simulink model "Buck_Converter_with_3ph_Full_Bridge_Rectifier"  (R2022b)
settings: Solver=VariableStepAuto  StartTime=0.0  StopTime=1.5  RelTol=1e-3
libraries: spsDiodeLib x7, spsSeriesRLCBranchLib x6, spsRMSLib x4, spsVoltageMeasurementLib x3, slpidlib x1, simulink x1, spsCurrentMeasurementLib x1, spsGroundLib x1, spsDCMachineLib x1, spsDCVoltageSourceLib x1, spsIGBTDiodeLib x1, spsPower3phInstantaneousLib x1
settings Model: Creator=meteh  LastModifiedBy=meteh
settings SolverCC: ZeroCrossAlgorithm=Adaptive
settings DebuggingCC: IgnoredZcDiagnostic=none

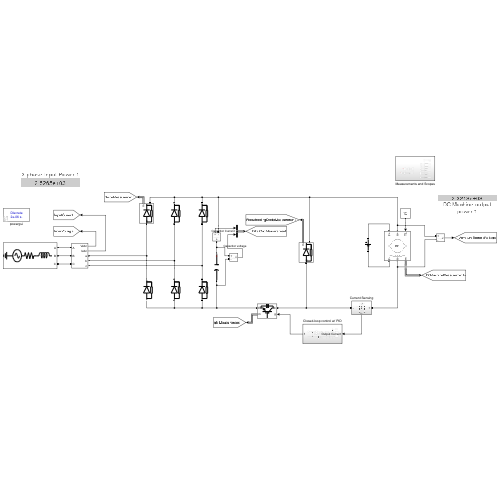
[thumbnail: Simulink's stored preview of the top-level diagram]
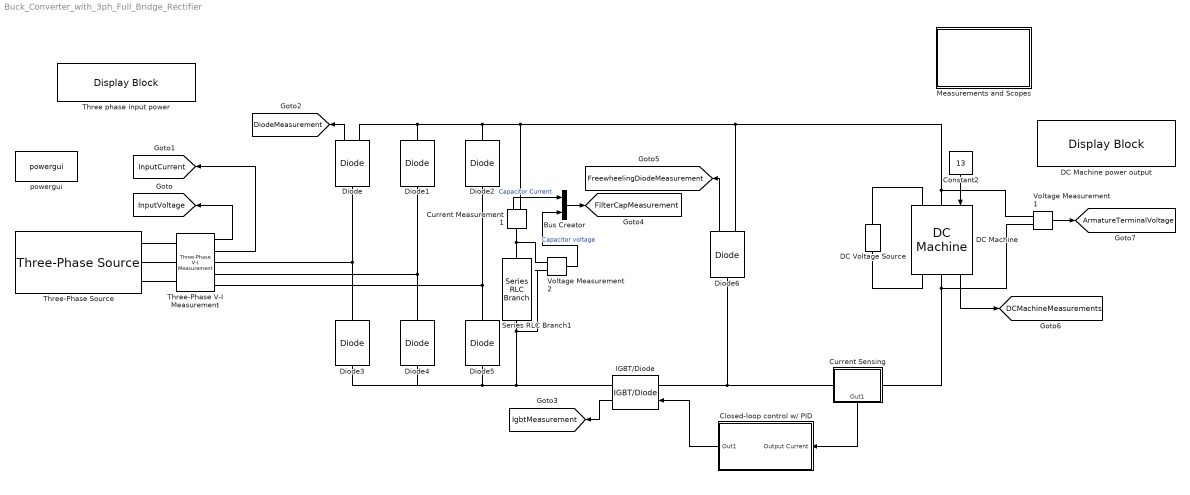
== system Buck_Converter_with_3ph_Full_Bridge_Rectifier ==
  Bus Creator : BusCreator  Inputs=2
  Closed-loop control w/ PID : Subsystem
  Constant2 : Constant  Value=13
  Current Measurement1 : spsCurrentMeasurementLib/Current Measurement  PhasorSimulation=off  OutputType=Complex  PSBequivalent=0
  Current Sensing : Subsystem
      settings: PortSchema="{\"entries\":[{\"content\":{\"sides\":[{\"content\":{\"connectorIds\":[\"LConn1\"]},\"type\":\"ConnectorPlacement.EquallySpacedRectSide\",\"uuid\":\"6fa835bd-a2a4-417c-aa91-2e27fd6635f1\"},{\"content\":{\"connectorIds\":[\"RConn1\"],\"side\":\"RIGHT\"},\"type\":\"ConnectorPlacement.EquallySpacedRectSide\",\"uuid\":\"e9586d19-de97-4ead-9c55-c2528cb3bc0e\"},{\"content\":{\"connectorIds\":[\"Out1\"],\"side\":\"TOP\"},\"type\":\"ConnectorPlacement.EquallySpacedRectSide\",\"uuid\":\"424d4a95-090a-4dbd-b56e-3f349dbd57f8\"}]},\"type\":\"ConnectorPlacement.EquallySpacedConnector\",\"uuid\":\"c618b47f-ea3e-4942-947b-44e1bd30c47a\"}],\"packageUris\":[\"http://schema.mathworks.com/mf0/Connector/R2020b\"],\"version\":\"1.0\"}"
  DC Machine : spsDCMachineLib/DC Machine  PresetModel=No  MechanicalLoad=Torque TL  FieldType=Wound  ShowDetailedParameters=on  MeasurementBus=off  RLa="[ 0.8  0.0125]"  RLf="[ 210  23]"  Laf=1  MachineConstant=Torque constant (N.m/A)  Ke=1.8  Kt=1.8  J=0.001  Bm=0.001  Tf=0.001  w0=0  Ifinit=0.952380952380952  TsPowergui=0  TsBlock=-1
  DC Machine power output : DisplayBlock  LabelPosition=Bottom  Transparency=1
  DC Voltage Source : spsDCVoltageSourceLib/DC Voltage Source  Amplitude=200  Measurements=None
  Diode : spsDiodeLib/Diode  Ron=0.001  Lon=0  Vf=0.8  IC=0  UseSnubber=0  Rs=500  Cs=250e-9  Measurements=on
  Diode{1..5} (5 alike) : spsDiodeLib/Diode  Ron=0.001  Lon=0  Vf=0.8  IC=0  UseSnubber=0  Rs=500  Cs=250e-9  Measurements=off
  Diode6 : spsDiodeLib/Diode  Ron=0.001  Lon=0  Vf=0.8  IC=0  UseSnubber=0  Rs=500  Cs=250e-9  Measurements=on
  IGBT/Diode : spsIGBTDiodeLib/IGBT//Diode  Ron=1e-3  Rs=1e5  Cs=inf  Measurements=on
  Measurements and Scopes : Subsystem
  Series RLC Branch1 : spsSeriesRLCBranchLib/Series RLC Branch  LConnTagsString=__new0  RConnTagsString=__new0  BranchType=C  Resistance=0.8  Inductance=12.5e-3  SetiL0=off  InitialCurrent=0  Capacitance=940e-6  Setx0=off  InitialVoltage=0  Measurements=None
  Three phase input power : DisplayBlock  Description=Three phase input power  Transparency=1  Layout=Fill available space
  Three-Phase V-I Measurement : spsThreePhaseVIMeasurementLib/Three-Phase V-I Measurement  VoltageMeasurement=phase-to-ground  SetLabelV=off  LabelV=Vabc  Vpu=off  VpuLL=off  CurrentMeasurement=yes  SetLabelI=off  LabelI=Iabc  Ipu=off  Pbase=100e6  Vbase=500e3  OutputType=Complex  PhasorSimulation=off  PSBequivalent=0
  Three-Phase Source : spsThreePhaseSourceLib/Three-Phase Source  InternalConnection=Yg  VoltagePhases=off  Voltage=133  PhaseAngle=0  Voltage_phases=[25e3 25e3 25e3]/sqrt(3)  PhaseAngles_phases=[0 -120 +120]  Frequency=50  NonIdealSource=on  SpecifyImpedance=off  Resistance=0.02  Inductance=2e-3  ShortCircuitLevel=100e6  BaseVoltage=25e3  XRratio=7  BusType=swing  Pref=10e3  Qref=0  Prefabc=[10e3, 10e3, 10e3]  Qrefabc=[0, 0, 0]  Qmin=-inf  Qmax=inf
  Voltage Measurement1 : spsVoltageMeasurementLib/Voltage Measurement  PhasorSimulation=off  OutputType=Complex  PSBequivalent=0
  Voltage Measurement2 : spsVoltageMeasurementLib/Voltage Measurement  PhasorSimulation=off  OutputType=Complex  PSBequivalent=0
  powergui : spspowerguiLib/powergui  Priority=1  SimulationMode=Discrete  SampleTime=2e-6  frequency=60  Iterations=50  frequencyindice=0  Pbase=100e6  ErrMax=1e-4  UnitsV=kV  UnitsW=MW  buscounter=0  FunctionMessages=off  echomessages=off  EnableUseOfTLC=off  CurrentSourceSwitches=off  DisableSnubberDevices=off  DisableRonSwitches=off  DisableVfSwitches=off  DisplayEquations=off  AutomaticDiscreteSolvers=off  SolverType=Tustin/Backward Euler (TBE)  Interpol=off  ExternalGateDelay=off  methode=off  Ts=100  x0status=blocks  SPID=on  SwTol=0  HookPort=off  NonlinearTolerance=1e-4  nMaxIteration=100  ContinueOnMaxIteration=off  RestoreLinks=warning  ResistiveCurrentMeasurement=off  Frange=[0:2:500]  Ylog=off  Xlog=on  ShowGrid=off  save=off  variable=ZData  structure=0  ZoomFFT=off  StartTime=0.0  cycles=1  DisplayStyle=1  fundamental=60  FreqAxis=off  MaxFrequency=1000  frequencyindicesteady=1  RmsSteady=1  display=off
  tag scope: ArmatureTerminalVoltage=global, DCMachineMeasurements=global, DiodeMeasurement=global, FilterCapMeasurement=global, FreewheelingDiodeMeasurement=global, IgbtMeasurement=global, InputCurrent=global, InputVoltage=global
  wires:
  Constant2/1 -> DC Machine/1
  Three-Phase V-I Measurement/2 -> [InputCurrent]
  Three-Phase V-I Measurement/1 -> [InputVoltage]
  Diode6/1 -> [FreewheelingDiodeMeasurement]
  Current Measurement1/1 -> Bus Creator/1  "Capacitor Current"
  Voltage Measurement2/1 -> Bus Creator/2  "Capacitor voltage"
  Bus Creator/1 -> [FilterCapMeasurement]
  DC Machine/1 -> [DCMachineMeasurements]
  Voltage Measurement1/1 -> [ArmatureTerminalVoltage]
  Diode/1 -> [DiodeMeasurement]
  IGBT/Diode/1 -> [IgbtMeasurement]
  Current Sensing/1(Out1) -> Closed-loop control w/ PID/1(Output Current)
  Closed-loop control w/ PID/1(Out1) -> IGBT/Diode/1
  connections:
  Diode3/RConn1 -- Three-Phase V-I Measurement/RConn1 -- Diode/LConn1
  Diode4/RConn1 -- Three-Phase V-I Measurement/RConn2 -- Diode1/LConn1
  Diode5/RConn1 -- Diode2/LConn1 -- Three-Phase V-I Measurement/RConn3
  Series RLC Branch1/RConn1 -- IGBT/Diode/RConn1 -- Diode3/LConn1 -- Diode4/LConn1 -- Diode5/LConn1 -- Voltage Measurement2/LConn2
  Three-Phase Source/RConn1 -- Three-Phase V-I Measurement/LConn1
  Three-Phase Source/RConn2 -- Three-Phase V-I Measurement/LConn2
  Three-Phase Source/RConn3 -- Three-Phase V-I Measurement/LConn3
  DC Voltage Source/RConn1 -- DC Machine/LConn2
  DC Machine/RConn2 -- DC Voltage Source/LConn1
  Current Measurement1/RConn1 -- Voltage Measurement1/LConn1 -- DC Machine/LConn1 -- Diode6/RConn1 -- Diode/RConn1 -- Diode1/RConn1 -- Diode2/RConn1
  Current Measurement1/LConn1 -- Series RLC Branch1/LConn1 -- Voltage Measurement2/LConn1
  DC Machine/RConn1 -- Current Sensing/LConn1 -- Voltage Measurement1/LConn2
  Diode6/LConn1 -- IGBT/Diode/LConn1 -- Current Sensing/RConn1

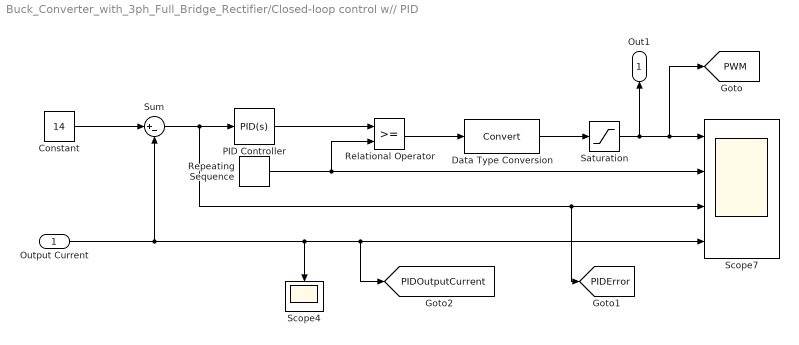
== system Buck_Converter_with_3ph_Full_Bridge_Rectifier/Closed-loop control w// PID ==
  Output Current : Inport
  Constant : Constant  Value=14
  Data Type Conversion : DataTypeConversion  OutMin=[0.01]  OutMax=[1]  SaturateOnIntegerOverflow=off  RndMeth=Floor
  PID Controller : slpidlib/PID Controller  Controller=PID  Form=Parallel  TimeDomain=Continuous-time  UseExternalTs=off  SampleTime=-1  IntegratorMethod=Forward Euler  FilterMethod=Forward Euler  ControllerParametersSource=internal  P=100  I=20  UseKiTs=off  D=1  N=100  UseFilter=on  TunerSelectOption=Transfer Function Based (PID Tuner App)  InitialConditionSource=internal  InitialConditionForIntegrator=0  InitialConditionForFilter=0  DifferentiatorICPrevScaledInput=0  ExternalReset=none  TrackingMode=off  Kt=1  LimitOutput=off  SatLimitsSource=internal  UpperSaturationLimit=inf  LowerSaturationLimit=-inf  LinearizeAsGain=on  AntiWindupMode=none  Kb=1  LimitIntegrator=off  UpperIntegratorSaturationLimit=inf  LowerIntegratorSaturationLimit=-inf  POutMin=[]  POutMax=[]  IOutMin=[]  IOutMax=[]  DOutMin=[]  DOutMax=[]  NOutMin=[]  NOutMax=[]  SumOutMin=[]  SumOutMax=[]  SaturationOutMin=[]  SaturationOutMax=[]  PParamMin=[]  PParamMax=[]  IParamMin=[]  IParamMax=[]  DParamMin=[]  DParamMax=[]  NParamMin=[]  NParamMax=[]  KbParamMin=[]  KbParamMax=[]  KtParamMin=[]  KtParamMax=[]  KbOutMin=[]  KbOutMax=[]  KtOutMin=[]  KtOutMax=[]  IntegratorOutMin=[]  IntegratorOutMax=[]  FilterOutMin=[]  FilterOutMax=[]  SumI1OutMin=[]  SumI1OutMax=[]  SumI2OutMin=[]  SumI2OutMax=[]  SumI3OutMin=[]  SumI3OutMax=[]  SumI4OutMin=[]  SumI4OutMax=[]  SumDOutMin=[]  SumDOutMax=[]  DifferentiatorOutMin=[]  DifferentiatorOutMax=[]  FilterDiffOutCoefMin=[]  FilterDiffOutCoefMax=[]  ReciprocalOutMin=[]  ReciprocalOutMax=[]  SumDenOutMin=[]  SumDenOutMax=[]  SumNumOutMin=[]  SumNumOutMax=[]  DivideOutMin=[]  DivideOutMax=[]  UdiffTsProdOutMin=[]  UdiffTsProdOutMax=[]  NTsProdOutMin=[]  NTsProdOutMax=[]  UintegralTsProdOutMin=[]  UintegralTsProdOutMax=[]  UngainTsProdOutMin=[]  UngainTsProdOutMax=[]  ClampingZeroOutDataTypeStr=Inherit: Inherit via back propagation  ClampingZeroOutMin=[]  ClampingZeroOutMax=[]  FilterDenConstantOutDataTypeStr=Inherit: Inherit via back propagation  FilterDenConstantOutMin=[]  FilterDenConstantOutMax=[]  PCopyOutDataTypeStr=Inherit: Inherit via back propagation  PCopyOutMin=[]  PCopyOutMax=[]  NCopyOutDataTypeStr=Inherit: Inherit via back propagation  NCopyOutMin=[]  NCopyOutMax=[]  IntegratorContinuousStateAttributes=''  IntegratorStateMustResolveToSignalObject=off  IntegratorRTWStateStorageClass=Auto  FilterContinuousStateAttributes=''  FilterStateMustResolveToSignalObject=off  FilterRTWStateStorageClass=Auto  ParallelPVariant=InternalParameters  IdealPVariant=Disabled  IVariant=InternalParameters  DVariant=InternalParameters  IntegratorVariant=Continuous  SatVariant=Disabled  AWVariant=Passthrough  PCopyVariant=Disabled  TRVariant=Disabled  FdbkBlocksVariant=Forward  IdealPFdbkVariant=Disabled  SatFdbkVariant=Disabled  DerivativeFilterVariant=ContFilter  NVariant=InternalParameters  NCopyVariant=Disabled  FilterICVariant=InternalICsFilter  IntegratorICVariant=InternalICs  ExternalResetVariant=Disabled  TRSumVariant=Passthrough  SumFdbkVariant=Disabled  SumVariant=Sum_PID  TsampFilterVariant=InternalTs  TsampNgainVariant=Passthrough  TsampIntegralVariant=Passthrough  ExternalSaturationOutDataTypeStr=Inherit: Same as second input
  Relational Operator : RelationalOperator  OutDataTypeStr=boolean  RndMeth=Simplest  InputSameDT=off
  Repeating Sequence : simulink/Sources/Repeating Sequence  rep_seq_t=[0 5e-3]  rep_seq_y=[0 15]
  Saturation : Saturate  UpperLimit=1  LowerLimit=0
  Scope4 : Scope
  Scope7 : Scope  NumInputPorts=4
  Sum : Sum  Inputs=|+-
  Out1 : Outport
  tag scope: PIDError=global, PIDOutputCurrent=global, PWM=global
  wires:
  Repeating Sequence/1 -> Scope7/2, Relational Operator/2
  Saturation/1 -> Out1/1, [PWM], Scope7/1
  Output Current/1 -> Scope7/4, [PIDOutputCurrent], Scope4/1, Sum/2
  Sum/1 -> [PIDError], Scope7/3, PID Controller/1
  Data Type Conversion/1 -> Saturation/1
  PID Controller/1 -> Relational Operator/1
  Constant/1 -> Sum/1
  Relational Operator/1 -> Data Type Conversion/1

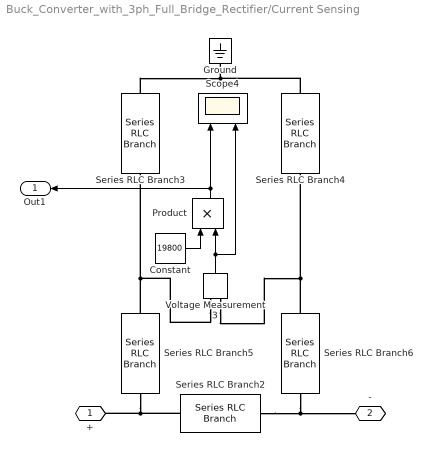
== system Buck_Converter_with_3ph_Full_Bridge_Rectifier/Current Sensing ==
  Constant : Constant  Value=19800
  Ground : spsGroundLib/Ground  LConnTagsString=a
  Product : Product
  Scope4 : Scope  NumInputPorts=2
  Series RLC Branch2 : spsSeriesRLCBranchLib/Series RLC Branch  LConnTagsString=__new0  RConnTagsString=__new0  BranchType=R  Resistance=0.005  Inductance=12.5e-3  SetiL0=off  InitialCurrent=0  Capacitance=940e-6  Setx0=off  InitialVoltage=0  Measurements=None
  Series RLC Branch3 : spsSeriesRLCBranchLib/Series RLC Branch  LConnTagsString=__new0  RConnTagsString=__new0  BranchType=R  Resistance=500  Inductance=12.5e-3  SetiL0=off  InitialCurrent=0  Capacitance=940e-6  Setx0=off  InitialVoltage=0  Measurements=None
  Series RLC Branch4 : spsSeriesRLCBranchLib/Series RLC Branch  LConnTagsString=__new0  RConnTagsString=__new0  BranchType=R  Resistance=500  Inductance=12.5e-3  SetiL0=off  InitialCurrent=0  Capacitance=940e-6  Setx0=off  InitialVoltage=0  Measurements=None
  Series RLC Branch5 : spsSeriesRLCBranchLib/Series RLC Branch  LConnTagsString=__new0  RConnTagsString=__new0  BranchType=R  Resistance=49e3  Inductance=12.5e-3  SetiL0=off  InitialCurrent=0  Capacitance=940e-6  Setx0=off  InitialVoltage=0  Measurements=None
  Series RLC Branch6 : spsSeriesRLCBranchLib/Series RLC Branch  LConnTagsString=__new0  RConnTagsString=__new0  BranchType=R  Resistance=49e3  Inductance=12.5e-3  SetiL0=off  InitialCurrent=0  Capacitance=940e-6  Setx0=off  InitialVoltage=0  Measurements=None
  Voltage Measurement3 : spsVoltageMeasurementLib/Voltage Measurement  PhasorSimulation=off  OutputType=Complex  PSBequivalent=0
  + : PMIOPort  Side=Left
  - : PMIOPort  Port=2  Side=Right
  Out1 : Outport
  wires:
  Constant/1 -> Product/1
  Product/1 -> Scope4/1, Out1/1
  Voltage Measurement3/1 -> Scope4/2, Product/2
  connections:
  Series RLC Branch3/RConn1 -- Ground/LConn1 -- Series RLC Branch4/RConn1
  Series RLC Branch5/RConn1 -- Series RLC Branch3/LConn1 -- Voltage Measurement3/LConn1
  Series RLC Branch6/RConn1 -- Voltage Measurement3/LConn2 -- Series RLC Branch4/LConn1
  Series RLC Branch6/LConn1 -- Series RLC Branch2/LConn1 -- -/RConn1
  Series RLC Branch5/LConn1 -- Series RLC Branch2/RConn1 -- +/RConn1

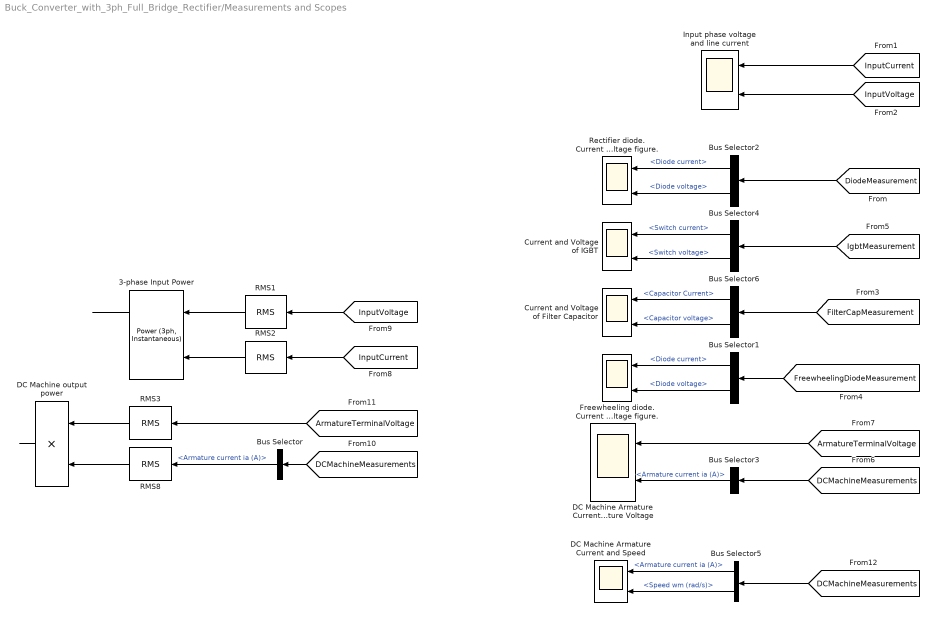
== system Buck_Converter_with_3ph_Full_Bridge_Rectifier/Measurements and Scopes ==
  3-phase Input Power : spsPower3phInstantaneousLib/Power (3ph, Instantaneous)
  Bus Selector : BusSelector  OutputSignals=Armature current ia (A)
  Bus Selector1 : BusSelector  OutputSignals=Diode current,Diode voltage
  Bus Selector2 : BusSelector  OutputSignals=Diode current,Diode voltage
  Bus Selector3 : BusSelector  OutputSignals=Armature current ia (A)
  Bus Selector4 : BusSelector  OutputSignals=Switch current,Switch voltage
  Bus Selector5 : BusSelector  OutputSignals=Armature current ia (A),Speed wm (rad/s)
  Bus Selector6 : BusSelector  OutputSignals=Capacitor Current,Capacitor voltage
  Current and Voltage of Filter Capacitor : Scope  NumInputPorts=2
  Current and Voltage of IGBT : Scope  NumInputPorts=2
  DC Machine Armature Current and Armature Voltage : Scope  NumInputPorts=2
  DC Machine Armature Current and Speed : Scope  NumInputPorts=2
  DC Machine output power : Product
  Freewheeling diode. Current and Voltage figure. : Scope  NumInputPorts=2
  Input phase voltage and line current : Scope  NumInputPorts=2
  RMS1 : spsRMSLib/RMS  TrueRMS=on  Freq=50  RMSInit=0  Ts=0
  RMS2 : spsRMSLib/RMS  TrueRMS=on  Freq=50  RMSInit=0  Ts=0
  RMS3 : spsRMSLib/RMS  TrueRMS=on  Freq=50  RMSInit=0  Ts=0
  RMS8 : spsRMSLib/RMS  TrueRMS=on  Freq=60  RMSInit=0  Ts=0
  Rectifier diode. Current and voltage figure. : Scope  NumInputPorts=2
  wires:
  Bus Selector/1 -> RMS8/1  "<Armature current ia (A)>"
  [FreewheelingDiodeMeasurement] -> Bus Selector1/1
  Bus Selector1/1 -> Freewheeling diode. Current and Voltage figure./1  "<Diode current>"
  Bus Selector1/2 -> Freewheeling diode. Current and Voltage figure./2  "<Diode voltage>"
  [DiodeMeasurement] -> Bus Selector2/1
  Bus Selector2/1 -> Rectifier diode. Current and voltage figure./1  "<Diode current>"
  Bus Selector2/2 -> Rectifier diode. Current and voltage figure./2  "<Diode voltage>"
  [ArmatureTerminalVoltage] -> DC Machine Armature Current and Armature Voltage/1
  [DCMachineMeasurements] -> Bus Selector3/1
  Bus Selector3/1 -> DC Machine Armature Current and Armature Voltage/2  "<Armature current ia (A)>"
  [IgbtMeasurement] -> Bus Selector4/1
  Bus Selector4/1 -> Current and Voltage of IGBT/1  "<Switch current>"
  Bus Selector4/2 -> Current and Voltage of IGBT/2  "<Switch voltage>"
  [DCMachineMeasurements] -> Bus Selector/1
  [DCMachineMeasurements] -> Bus Selector5/1
  Bus Selector5/1 -> DC Machine Armature Current and Speed/1  "<Armature current ia (A)>"
  Bus Selector5/2 -> DC Machine Armature Current and Speed/2  "<Speed wm (rad/s)>"
  Bus Selector6/2 -> Current and Voltage of Filter Capacitor/2  "<Capacitor voltage>"
  Bus Selector6/1 -> Current and Voltage of Filter Capacitor/1  "<Capacitor Current>"
  [FilterCapMeasurement] -> Bus Selector6/1
  [InputCurrent] -> Input phase voltage and line current/1
  [InputVoltage] -> Input phase voltage and line current/2
  3-phase Input Power/1 -> ?
  [ArmatureTerminalVoltage] -> RMS3/1
  [InputVoltage] -> RMS1/1
  [InputCurrent] -> RMS2/1
  RMS3/1 -> DC Machine output power/1
  RMS1/1 -> 3-phase Input Power/1
  RMS2/1 -> 3-phase Input Power/2
  RMS8/1 -> DC Machine output power/2
  DC Machine output power/1 -> ?
